simulink model "waypoint_navigation"  (R2025a)
settings: Solver=FixedStepAuto  StartTime=0.0  StopTime=25  FixedStep=0.05  RelTol=1e-3
values from neighbouring files (symbols this model uses):
  L = 0.40000    (= 0.4)    [DiffDriveValue.m]
  R = 0.05663    [DiffDriveValue.m]
undefined symbols (not defined in the file or in its folder): DiscIntNeverNeededParam
libraries: arduinolib x6, simulink x4, slpidlib x2, robotalgslib x1, mobileRoboticsLib x1
settings Model: Creator=ASUS  LastModifiedBy=ASUS
settings SolverCC: EnableFixedStepZeroCrossing=on

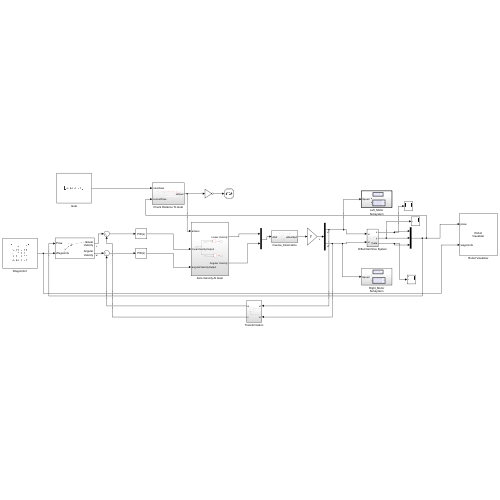
[thumbnail: Simulink's stored preview of the top-level diagram]
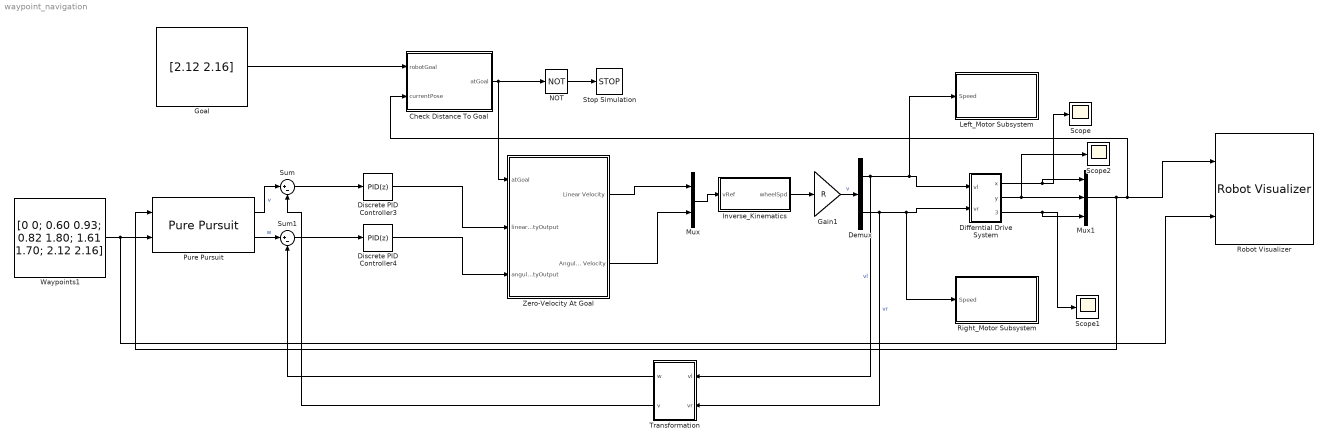
== system waypoint_navigation ==
  Check Distance To Goal : Subsystem
  Demux : Demux  Outputs=2
  Differntial Drive System : Subsystem
  Discrete PID Controller3 : slpidlib/PID Controller  Controller=PID  Form=Parallel  TimeDomain=Discrete-time  UseExternalTs=off  SampleTime=-1  IntegratorMethod=Forward Euler  FilterMethod=Forward Euler  ControllerParametersSource=internal  P=0.053595  I=0.10445  UseKiTs=on  D=0  UseExternalDerivativeSource=off  N=100  UseFilter=on  TunerSelectOption=Frequency Response Based  InitialConditionSource=internal  InitialConditionForIntegrator=0  InitialConditionForFilter=0  DifferentiatorICPrevScaledInput=0  ExternalReset=none  TrackingMode=off  Kt=1  LimitOutput=off  SatLimitsSource=internal  UpperSaturationLimit=inf  LowerSaturationLimit=-inf  LinearizeAsGain=off  AntiWindupMode=none  Kb=1  LimitIntegrator=off  UpperIntegratorSaturationLimit=inf  LowerIntegratorSaturationLimit=-inf  POutMin=[]  POutMax=[]  IOutMin=[]  IOutMax=[]  DOutMin=[]  DOutMax=[]  NOutMin=[]  NOutMax=[]  SumOutMin=[]  SumOutMax=[]  SaturationOutMin=[]  SaturationOutMax=[]  PParamMin=[]  PParamMax=[]  IParamMin=[]  IParamMax=[]  DParamMin=[]  DParamMax=[]  NParamMin=[]  NParamMax=[]  KbParamMin=[]  KbParamMax=[]  KtParamMin=[]  KtParamMax=[]  KbOutMin=[]  KbOutMax=[]  KtOutMin=[]  KtOutMax=[]  IntegratorOutMin=[]  IntegratorOutMax=[]  FilterOutMin=[]  FilterOutMax=[]  SumI1OutMin=[]  SumI1OutMax=[]  SumI2OutMin=[]  SumI2OutMax=[]  SumI3OutMin=[]  SumI3OutMax=[]  SumI4OutMin=[]  SumI4OutMax=[]  SumDOutMin=[]  SumDOutMax=[]  DifferentiatorOutMin=[]  DifferentiatorOutMax=[]  FilterDiffOutCoefMin=[]  FilterDiffOutCoefMax=[]  ReciprocalOutMin=[]  ReciprocalOutMax=[]  SumDenOutMin=[]  SumDenOutMax=[]  SumNumOutMin=[]  SumNumOutMax=[]  DivideOutMin=[]  DivideOutMax=[]  UdiffTsProdOutMin=[]  UdiffTsProdOutMax=[]  NTsProdOutMin=[]  NTsProdOutMax=[]  UintegralTsProdOutMin=[]  UintegralTsProdOutMax=[]  UngainTsProdOutMin=[]  UngainTsProdOutMax=[]  ClampingZeroOutDataTypeStr=Inherit: Inherit via back propagation  ClampingZeroOutMin=[]  ClampingZeroOutMax=[]  FilterDenConstantOutDataTypeStr=Inherit: Inherit via back propagation  FilterDenConstantOutMin=[]  FilterDenConstantOutMax=[]  PCopyOutDataTypeStr=Inherit: Inherit via back propagation  PCopyOutMin=[]  PCopyOutMax=[]  NCopyOutDataTypeStr=Inherit: Inherit via back propagation  NCopyOutMin=[]  NCopyOutMax=[]  IntegratorContinuousStateAttributes=''  IntegratorStateMustResolveToSignalObject=off  IntegratorRTWStateStorageClass=Auto  FilterContinuousStateAttributes=''  FilterStateMustResolveToSignalObject=off  FilterRTWStateStorageClass=Auto  ParallelPVariant=InternalParameters  IdealPVariant=Disabled  IVariant=InternalParameters  DVariant=InternalParameters  IntegratorVariant=Discrete  SatVariant=Disabled  AWVariant=Passthrough  PCopyVariant=Disabled  TRVariant=Disabled  FdbkBlocksVariant=Forward  IdealPFdbkVariant=Disabled  SatFdbkVariant=Disabled  DerivativeFilterVariant=ForwardEulerFilter  NVariant=InternalParameters  NCopyVariant=Disabled  FilterICVariant=InternalICsFilter  IntegratorICVariant=InternalICs  ExternalResetVariant=Disabled  TRSumVariant=Passthrough  SumFdbkVariant=Disabled  SumVariant=Sum_PID  TsampFilterVariant=InternalTs  TsampNgainVariant=Passthrough  TsampIntegralVariant=Disabled_SignalSpec  ExternalSaturationOutDataTypeStr=Inherit: Same as second input  DerivativeSourceVariant=ErrorSignal  PreIntVariant=InternalPreInt
      settings: LibrarySourceBlock=simulink/Discrete/Discrete PID Controller
  Discrete PID Controller4 : slpidlib/PID Controller  Controller=PID  Form=Parallel  TimeDomain=Discrete-time  UseExternalTs=off  SampleTime=-1  IntegratorMethod=Forward Euler  FilterMethod=Forward Euler  ControllerParametersSource=internal  P=0  I=0.92615  UseKiTs=on  D=0  UseExternalDerivativeSource=off  N=100  UseFilter=on  TunerSelectOption=Frequency Response Based  InitialConditionSource=internal  InitialConditionForIntegrator=0  InitialConditionForFilter=0  DifferentiatorICPrevScaledInput=0  ExternalReset=none  TrackingMode=off  Kt=1  LimitOutput=off  SatLimitsSource=internal  UpperSaturationLimit=inf  LowerSaturationLimit=-inf  LinearizeAsGain=off  AntiWindupMode=none  Kb=1  LimitIntegrator=off  UpperIntegratorSaturationLimit=inf  LowerIntegratorSaturationLimit=-inf  POutMin=[]  POutMax=[]  IOutMin=[]  IOutMax=[]  DOutMin=[]  DOutMax=[]  NOutMin=[]  NOutMax=[]  SumOutMin=[]  SumOutMax=[]  SaturationOutMin=[]  SaturationOutMax=[]  PParamMin=[]  PParamMax=[]  IParamMin=[]  IParamMax=[]  DParamMin=[]  DParamMax=[]  NParamMin=[]  NParamMax=[]  KbParamMin=[]  KbParamMax=[]  KtParamMin=[]  KtParamMax=[]  KbOutMin=[]  KbOutMax=[]  KtOutMin=[]  KtOutMax=[]  IntegratorOutMin=[]  IntegratorOutMax=[]  FilterOutMin=[]  FilterOutMax=[]  SumI1OutMin=[]  SumI1OutMax=[]  SumI2OutMin=[]  SumI2OutMax=[]  SumI3OutMin=[]  SumI3OutMax=[]  SumI4OutMin=[]  SumI4OutMax=[]  SumDOutMin=[]  SumDOutMax=[]  DifferentiatorOutMin=[]  DifferentiatorOutMax=[]  FilterDiffOutCoefMin=[]  FilterDiffOutCoefMax=[]  ReciprocalOutMin=[]  ReciprocalOutMax=[]  SumDenOutMin=[]  SumDenOutMax=[]  SumNumOutMin=[]  SumNumOutMax=[]  DivideOutMin=[]  DivideOutMax=[]  UdiffTsProdOutMin=[]  UdiffTsProdOutMax=[]  NTsProdOutMin=[]  NTsProdOutMax=[]  UintegralTsProdOutMin=[]  UintegralTsProdOutMax=[]  UngainTsProdOutMin=[]  UngainTsProdOutMax=[]  ClampingZeroOutDataTypeStr=Inherit: Inherit via back propagation  ClampingZeroOutMin=[]  ClampingZeroOutMax=[]  FilterDenConstantOutDataTypeStr=Inherit: Inherit via back propagation  FilterDenConstantOutMin=[]  FilterDenConstantOutMax=[]  PCopyOutDataTypeStr=Inherit: Inherit via back propagation  PCopyOutMin=[]  PCopyOutMax=[]  NCopyOutDataTypeStr=Inherit: Inherit via back propagation  NCopyOutMin=[]  NCopyOutMax=[]  IntegratorContinuousStateAttributes=''  IntegratorStateMustResolveToSignalObject=off  IntegratorRTWStateStorageClass=Auto  FilterContinuousStateAttributes=''  FilterStateMustResolveToSignalObject=off  FilterRTWStateStorageClass=Auto  ParallelPVariant=InternalParameters  IdealPVariant=Disabled  IVariant=InternalParameters  DVariant=InternalParameters  IntegratorVariant=Discrete  SatVariant=Disabled  AWVariant=Passthrough  PCopyVariant=Disabled  TRVariant=Disabled  FdbkBlocksVariant=Forward  IdealPFdbkVariant=Disabled  SatFdbkVariant=Disabled  DerivativeFilterVariant=ForwardEulerFilter  NVariant=InternalParameters  NCopyVariant=Disabled  FilterICVariant=InternalICsFilter  IntegratorICVariant=InternalICs  ExternalResetVariant=Disabled  TRSumVariant=Passthrough  SumFdbkVariant=Disabled  SumVariant=Sum_PID  TsampFilterVariant=InternalTs  TsampNgainVariant=Passthrough  TsampIntegralVariant=Disabled_SignalSpec  ExternalSaturationOutDataTypeStr=Inherit: Same as second input  DerivativeSourceVariant=ErrorSignal  PreIntVariant=InternalPreInt
      settings: LibrarySourceBlock=simulink/Discrete/Discrete PID Controller
  Gain1 : Gain  Gain=R
  Goal : Constant  Value=[2.12 2.16]
  Inverse_Kinematics : Subsystem
  Left_Motor Subsystem : Subsystem  TreatAsAtomicUnit=on
  Mux : Mux  Inputs=2
  Mux1 : Mux  Inputs=3
  NOT : Logic  Operator=NOT  IconShape=distinctive  AllPortsSameDT=off  OutDataTypeStr=boolean
  Pure Pursuit : robotalgslib/Pure Pursuit  DesiredLinearVelocityPort=off  DesiredLinearVelocity=0.2  MaxAngularVelocity=0.7  LookaheadDistancePort=off  LookaheadDistance=0.35  TargetDirPort=off  SimulateUsing=Interpreted execution
      settings: LibrarySourceBlock=navlib/Control Algorithms/Pure Pursuit
  Right_Motor Subsystem : Subsystem
  Robot Visualizer : mobileRoboticsLib/Environments/Robot Visualizer  Priority=99  robotRadius=R  showTrajectory=on  hasWaypoints=on  hasLidar=off  sensorOffset=[ 0 0 ]  scanAngles=0  hasObjDetector=off  objDetectorOffset=[ 0, 0 ]  objDetectorAngle=0  objDetectorFOV=0  objDetectorMaxRange=0  objectColors=0  objectMarkers=s
  Scope : Scope
      settings: ActiveDisplayYMinimum=-0.35887  ActiveDisplayYMaximum=3.22985
  Scope1 : Scope
      settings: ActiveDisplayYMinimum=-0.77117  ActiveDisplayYMaximum=1.83569  DataLoggingVariableName=ScopeData4
  Scope2 : Scope
      settings: ActiveDisplayYMinimum=-0.39056  ActiveDisplayYMaximum=3.51506  DataLoggingVariableName=ScopeData3
  Stop Simulation : Stop
  Sum : Sum  Inputs=|+-
  Sum1 : Sum  Inputs=|+-
  Transformation : Subsystem
  Waypoints1 : Constant  Value=[0 0; 0.60 0.93; 0.82 1.80; 1.61 1.70; 2.12 2.16]
  Zero-Velocity At Goal : Subsystem
  wires:
  NOT/1 -> Stop Simulation/1
  Demux/1 -> Left_Motor Subsystem/1(Speed), Differntial Drive System/1(vl), Transformation/1(vl)  "vl"
  Mux1/1 -> Check Distance To Goal/2(currentPose), Robot Visualizer/1, Pure Pursuit/1
  Demux/2 -> Right_Motor Subsystem/1(Speed), Differntial Drive System/2(vr), Transformation/2(vr)  "vr"
  Differntial Drive System/2(y) -> Mux1/2, Scope2/1
  Sum/1 -> Discrete PID Controller3/1
  Gain1/1 -> Demux/1  "v"
  Pure Pursuit/2 -> Sum1/1  "w"
  Discrete PID Controller4/1 -> Zero-Velocity At Goal/3(angularVelocityOutput)
  Inverse_Kinematics/1(wheelSpd) -> Gain1/1
  Waypoints1/1 -> Robot Visualizer/2, Pure Pursuit/2
  Sum1/1 -> Discrete PID Controller4/1
  Check Distance To Goal/1(atGoal) -> Zero-Velocity At Goal/1(atGoal), NOT/1
  Transformation/1(w) -> Sum1/2
  Differntial Drive System/1(x) -> Mux1/1, Scope/1
  Goal/1 -> Check Distance To Goal/1(robotGoal)
  Transformation/2(v) -> Sum/2
  Pure Pursuit/1 -> Sum/1  "v"
  Zero-Velocity At Goal/2(Angular Velocity) -> Mux/2
  Differntial Drive System/3(theta) -> Mux1/3, Scope1/1
  Zero-Velocity At Goal/1(Linear Velocity) -> Mux/1
  Mux/1 -> Inverse_Kinematics/1(vRef)
  Discrete PID Controller3/1 -> Zero-Velocity At Goal/2(linearVelocityOutput)

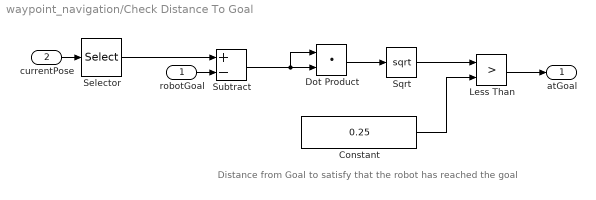
== system waypoint_navigation/Check Distance To Goal ==
  note: Distance from Goal to satisfy that the robot has reached the goal
  robotGoal : Inport
  currentPose : Inport  Port=2
  Constant : Constant  Value=0.25
  Dot Product : DotProduct  OutDataTypeStr=Inherit: Inherit via internal rule
  Less Than : RelationalOperator  Operator=>  OutDataTypeStr=boolean  RndMeth=Simplest  InputSameDT=off
  Selector : Selector  InputPortWidth=3  IndexOptions=Index vector (dialog)  Indices=[1 2]  OutputSizes=1
  Sqrt : Sqrt
  Subtract : Sum  Inputs=+-
  atGoal : Outport
  wires:
  robotGoal/1 -> Subtract/2
  Dot Product/1 -> Sqrt/1
  Constant/1 -> Less Than/2
  currentPose/1 -> Selector/1
  Less Than/1 -> atGoal/1
  Sqrt/1 -> Less Than/1
  Subtract/1 -> Dot Product/1, Dot Product/2
  Selector/1 -> Subtract/1

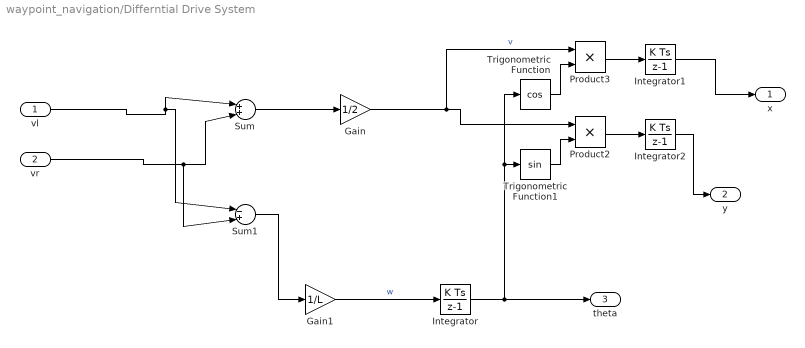
== system waypoint_navigation/Differntial Drive System ==
  vl : Inport
  vr : Inport  Port=2
  Gain : Gain  Gain=1/2
  Gain1 : Gain  Gain=1/L
  Integrator : DiscreteIntegrator  SampleTime=0.5  ICPrevOutput=DiscIntNeverNeededParam  ICPrevScaledInput=DiscIntNeverNeededParam  mask(DiscretizedDiscreteIntegrator){}
      mask init:
      | %zoh
  Integrator1 : DiscreteIntegrator  SampleTime=0.5  ICPrevOutput=DiscIntNeverNeededParam  ICPrevScaledInput=DiscIntNeverNeededParam  mask(DiscretizedDiscreteIntegrator){}
      mask init:
      | %zoh
  Integrator2 : DiscreteIntegrator  SampleTime=0.5  ICPrevOutput=DiscIntNeverNeededParam  ICPrevScaledInput=DiscIntNeverNeededParam  mask(DiscretizedDiscreteIntegrator){}
      mask init:
      | %zoh
  Product2 : Product
  Product3 : Product
  Sum : Sum  Inputs=|++|
  Sum1 : Sum  Inputs=|-+|
  Trigonometric Function : Trigonometry  Operator=cos
  Trigonometric Function1 : Trigonometry
  x : Outport
  y : Outport  Port=2
  theta : Outport  Port=3
  wires:
  Integrator1/1 -> x/1
  Integrator2/1 -> y/1
  Sum/1 -> Gain/1
  Product3/1 -> Integrator1/1
  Gain/1 -> Product2/1, Product3/1  "v"
  Integrator/1 -> Trigonometric Function1/1, Trigonometric Function/1, theta/1
  Gain1/1 -> Integrator/1  "w"
  vl/1 -> Sum1/1, Sum/1
  Sum1/1 -> Gain1/1
  Trigonometric Function1/1 -> Product2/2
  Trigonometric Function/1 -> Product3/2
  Product2/1 -> Integrator2/1
  vr/1 -> Sum/2, Sum1/2

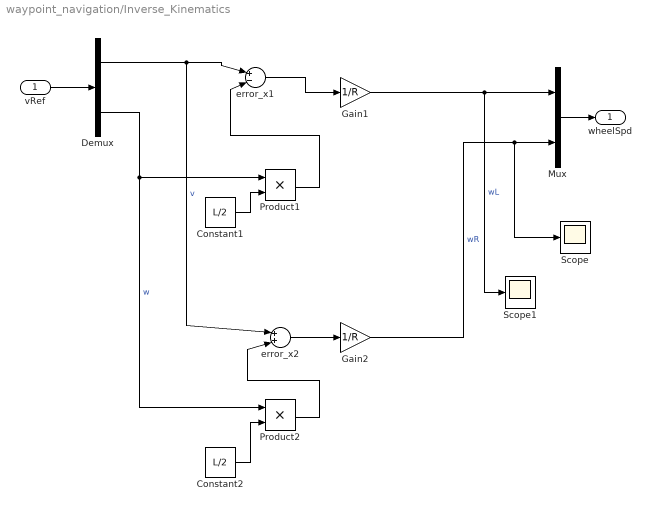
== system waypoint_navigation/Inverse_Kinematics ==
  vRef : Inport
  Constant1 : Constant  Value=L/2
  Constant2 : Constant  Value=L/2
  Demux : Demux  Outputs=2
  Gain1 : Gain  Gain=1/R
  Gain2 : Gain  Gain=1/R
  Mux : Mux  Inputs=2
  Product1 : Product
  Product2 : Product
  Scope : Scope
      settings: ActiveDisplayYMinimum=48.80275  ActiveDisplayYMaximum=68.80275
  Scope1 : Scope
      settings: ActiveDisplayYMinimum=37.14815  ActiveDisplayYMaximum=57.14815  DataLoggingVariableName=ScopeData2
  error_x1 : Sum  Inputs=|+-|
  error_x2 : Sum  Inputs=|++|
  wheelSpd : Outport  Unit=rad/s  VectorParamsAs1DForOutWhenUnconnected=off
  wires:
  Gain1/1 -> Scope1/1, Mux/1  "wL"
  Product1/1 -> error_x1/2
  Mux/1 -> wheelSpd/1
  Product2/1 -> error_x2/2
  Demux/2 -> Product2/1, Product1/1  "w"
  Constant1/1 -> Product1/2
  error_x1/1 -> Gain1/1
  Gain2/1 -> Mux/2, Scope/1  "wR"
  Demux/1 -> error_x1/1, error_x2/1  "v"
  error_x2/1 -> Gain2/1
  Constant2/1 -> Product2/2
  vRef/1 -> Demux/1

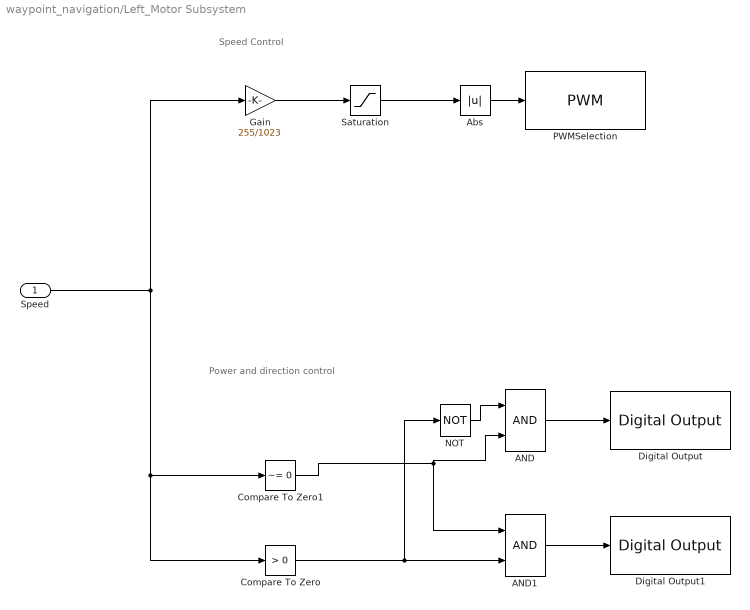
== system waypoint_navigation/Left_Motor Subsystem ==
  note: Power and direction control
  note: Speed Control
  Speed : Inport
  AND : Logic  IconShape=distinctive  AllPortsSameDT=off  OutDataTypeStr=boolean
  AND1 : Logic  IconShape=distinctive  AllPortsSameDT=off  OutDataTypeStr=boolean
  Abs : Abs  SaturateOnIntegerOverflow=off
  Compare To Zero : simulink/Logic and Bit Operations/Compare To Zero  relop=>  OutDataTypeStr=boolean
  Compare To Zero1 : simulink/Logic and Bit Operations/Compare To Zero  relop=~=  OutDataTypeStr=boolean
  Digital Output : arduinolib/Digital Output  pinNumber=5  Direction=output  blockPlatform=arduino
      settings: LibrarySourceBlock=arduinolib/L293D DC Motor/Digital Output
  Digital Output1 : arduinolib/Digital Output  pinNumber=9  Direction=output  blockPlatform=arduino
      settings: LibrarySourceBlock=arduinolib/L293D DC Motor/Digital Output1
  Gain : Gain  Gain=255/1023
  NOT : Logic  Operator=NOT  IconShape=distinctive  AllPortsSameDT=off  OutDataTypeStr=boolean
  PWMSelection : arduinolib/PWM  pinNumber=3  frequencyType=Default  desiredFrequency=490.2  achievableFrequency=490.2
      settings: LibrarySourceBlock=arduinolib/L293D DC Motor/PWMSelection
  Saturation : Saturate  UpperLimit=255  LowerLimit=-255
  wires:
  Saturation/1 -> Abs/1
  Abs/1 -> PWMSelection/1
  NOT/1 -> AND/1
  AND/1 -> Digital Output/1
  Compare To Zero1/1 -> AND1/1, AND/2
  Compare To Zero/1 -> AND1/2, NOT/1
  Speed/1 -> Gain/1, Compare To Zero/1, Compare To Zero1/1
  Gain/1 -> Saturation/1
  AND1/1 -> Digital Output1/1

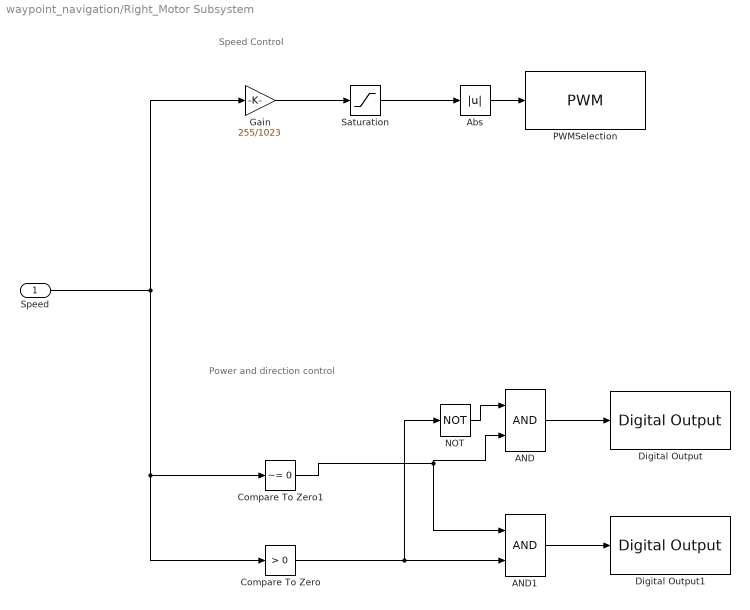
== system waypoint_navigation/Right_Motor Subsystem ==
  note: Power and direction control
  note: Speed Control
  Speed : Inport
  AND : Logic  IconShape=distinctive  AllPortsSameDT=off  OutDataTypeStr=boolean
  AND1 : Logic  IconShape=distinctive  AllPortsSameDT=off  OutDataTypeStr=boolean
  Abs : Abs  SaturateOnIntegerOverflow=off
  Compare To Zero : simulink/Logic and Bit Operations/Compare To Zero  relop=>  OutDataTypeStr=boolean
  Compare To Zero1 : simulink/Logic and Bit Operations/Compare To Zero  relop=~=  OutDataTypeStr=boolean
  Digital Output : arduinolib/Digital Output  pinNumber=6  Direction=output  blockPlatform=arduino
      settings: LibrarySourceBlock=arduinolib/L293D DC Motor/Digital Output
  Digital Output1 : arduinolib/Digital Output  pinNumber=10  Direction=output  blockPlatform=arduino
      settings: LibrarySourceBlock=arduinolib/L293D DC Motor/Digital Output1
  Gain : Gain  Gain=255/1023
  NOT : Logic  Operator=NOT  IconShape=distinctive  AllPortsSameDT=off  OutDataTypeStr=boolean
  PWMSelection : arduinolib/PWM  pinNumber=11  frequencyType=Default  desiredFrequency=490.2  achievableFrequency=490.2
      settings: LibrarySourceBlock=arduinolib/L293D DC Motor/PWMSelection
  Saturation : Saturate  UpperLimit=255  LowerLimit=-255
  wires:
  Saturation/1 -> Abs/1
  Abs/1 -> PWMSelection/1
  NOT/1 -> AND/1
  AND/1 -> Digital Output/1
  Compare To Zero1/1 -> AND1/1, AND/2
  Compare To Zero/1 -> AND1/2, NOT/1
  Speed/1 -> Gain/1, Compare To Zero/1, Compare To Zero1/1
  Gain/1 -> Saturation/1
  AND1/1 -> Digital Output1/1

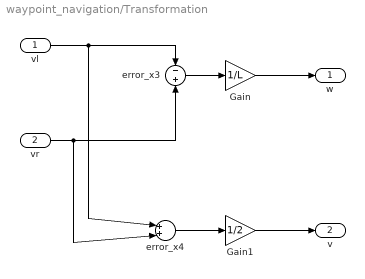
== system waypoint_navigation/Transformation ==
  vl : Inport
  vr : Inport  Port=2
  Gain : Gain  Gain=1/L
  Gain1 : Gain  Gain=1/2
  error_x3 : Sum  Inputs=-+
  error_x4 : Sum  Inputs=|++|
  w : Outport
  v : Outport  Port=2
  wires:
  vl/1 -> error_x4/1, error_x3/1
  vr/1 -> error_x4/2, error_x3/2
  error_x3/1 -> Gain/1
  Gain/1 -> w/1
  Gain1/1 -> v/1
  error_x4/1 -> Gain1/1

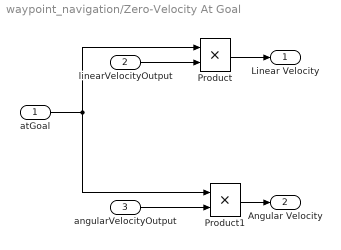
== system waypoint_navigation/Zero-Velocity At Goal ==
  atGoal : Inport
  linearVelocityOutput : Inport  Port=2
  angularVelocityOutput : Inport  Port=3
  Product : Product
  Product1 : Product
  Linear Velocity : Outport  OutDataTypeStr=double
  Angular Velocity : Outport  Port=2  OutDataTypeStr=double
  wires:
  atGoal/1 -> Product1/1, Product/1
  angularVelocityOutput/1 -> Product1/2
  linearVelocityOutput/1 -> Product/2
  Product/1 -> Linear Velocity/1
  Product1/1 -> Angular Velocity/1
